simulink model "carsimplesimulink"  (R2022b)
settings: Solver=FixedStepAuto  StartTime=0.0  StopTime=inf  FixedStep=0.05  RelTol=1e-3
libraries: robotlib x7
settings Model: Creator=sprinkle  LastModifiedBy=sprinkle
settings OptimizationCC: EnhancedBackFolding=on  PassReuseOutputArgsAs=Individual arguments  ZeroExternalMemoryAtStartup=off  ZeroInternalMemoryAtStartup=off  MaxStackSize=64  OptimizeBlockOrder=speed  DifferentSizesBufferReuse=on  OptimizationCustomize=off  EfficientTunableParamExpr=on
settings DebuggingCC: ParameterTunabilityLossMsg=error
settings HardwareCC: ProdBitPerPointer=32  ProdBitPerSizeT=32  ProdBitPerPtrDiffT=32  ProdLargestAtomicFloat=None  ProdIntDivRoundTo=Undefined  ProdEndianess=Unspecified  ProdWordSize=32  ProdHWDeviceType=Generic->Unspecified (assume 32-bit Generic)
settings SFSimCC: MATLABDynamicMemAlloc=off
settings RTWCC: Description=Embedded Coder  SystemTargetFile=ert.tlc  HardwareBoard=Robot Operating System (ROS)  TLCOptions="-aInlineSetEventsForThisBaseRateFcn=TLC_FALSE -aSuppressMultiTaskScheduler=TLC_FALSE  -aRateBasedStepFcn=0"  TemplateMakefile=ert_default_tmf  Toolchain=Catkin  TargetLang=C++
settings CodeAppCC: ForceParamTrailComments=on  IgnoreCustomStorageClasses=off  OperatorAnnotations=on  SimulinkDataObjDesc=on  SFDataObjDesc=on  InsertBlockDesc=on
settings ERTTargetCC: SupportContinuousTime=on

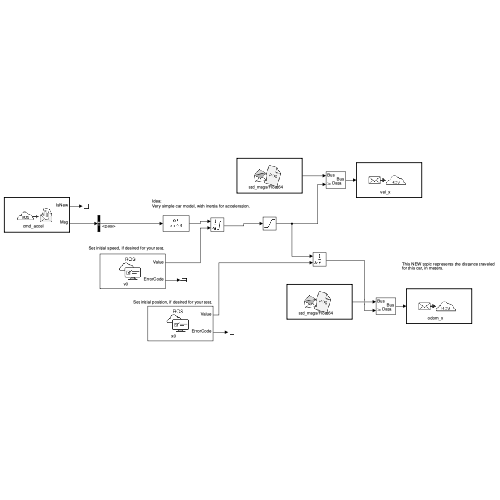
[thumbnail: Simulink's stored preview of the top-level diagram]
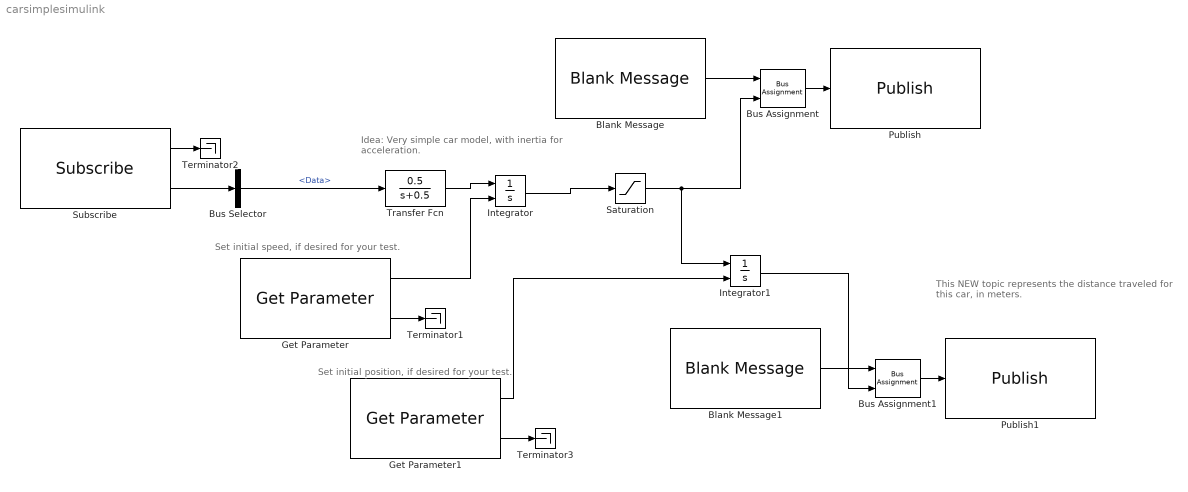
== system carsimplesimulink ==
  note: This NEW topic represents the distance traveled
      | for this car, in meters.
  note: Set initial speed, if desired for your test.
  note: Idea:
      | Very simple car model, with inertia for acceleration.
  note: Set initial position, if desired for your test.
  Blank Message : robotlib/Blank Message  messageClass=Message  entityType=std_msgs/Float64  messageType=std_msgs/Float64  SampleTime=inf  legacyBusStruct=off
      settings: LibrarySourceBlock=roslib/ROS/Blank Message
  Blank Message1 : robotlib/Blank Message  messageClass=Message  entityType=std_msgs/Float64  messageType=std_msgs/Float64  SampleTime=inf  legacyBusStruct=off
      settings: LibrarySourceBlock=roslib/ROS/Blank Message
  Bus Assignment : BusAssignment  AssignedSignals=Data
  Bus Assignment1 : BusAssignment  AssignedSignals=Data
  Bus Selector : BusSelector  OutputSignals=Data
  Get Parameter : robotlib/Get Parameter  ParameterSource=Specify your own  ParameterName=v0  ParameterType=double  ParameterMaxArrayLength=16  ParameterInitialValue=0.0  SampleTime=-1  ShowErrorCodeOutput=on  ModelName=carsimplesimulink  BlockId=ParamGet_carsimplesimulink_31
      settings: LibrarySourceBlock=roslib/ROS/Get Parameter
  Get Parameter1 : robotlib/Get Parameter  ParameterSource=Specify your own  ParameterName=x0  ParameterType=double  ParameterMaxArrayLength=16  ParameterInitialValue=0.0  SampleTime=-1  ShowErrorCodeOutput=on  ModelName=carsimplesimulink  BlockId=ParamGet_carsimplesimulink_37
      settings: LibrarySourceBlock=roslib/ROS/Get Parameter
  Integrator : Integrator  InitialConditionSource=external  LimitOutput=on  UpperSaturationLimit=40  LowerSaturationLimit=0
  Integrator1 : Integrator  InitialConditionSource=external
  Publish : robotlib/Publish  topicSource=Specify your own  topic=vel_x  messageType=std_msgs/Float64  legacyBusStruct=off  messageQueueLength=1
      settings: LibrarySourceBlock=roslib/ROS/Publish
  Publish1 : robotlib/Publish  topicSource=Specify your own  topic=odom_x  messageType=std_msgs/Float64  legacyBusStruct=off  messageQueueLength=1
      settings: LibrarySourceBlock=roslib/ROS/Publish
  Saturation : Saturate  UpperLimit=40  LowerLimit=0
  Subscribe : robotlib/Subscribe  topicSource=Specify your own  topic=cmd_accel  messageType=std_msgs/Float64  SampleTime=-1  legacyBusStruct=off  messageQueueLength=1
      settings: LibrarySourceBlock=roslib/ROS/Subscribe
  Terminator1 : Terminator
  Terminator2 : Terminator
  Terminator3 : Terminator
  Transfer Fcn : TransferFcn  Numerator=[0.5]  Denominator=[1 0.5]
  wires:
  Bus Selector/1 -> Transfer Fcn/1  "<Data>"
  Transfer Fcn/1 -> Integrator/1
  Subscribe/1 -> Terminator2/1
  Integrator/1 -> Saturation/1
  Blank Message/1 -> Bus Assignment/1
  Bus Assignment/1 -> Publish/1
  Subscribe/2 -> Bus Selector/1
  Saturation/1 -> Integrator1/1, Bus Assignment/2
  Get Parameter/1 -> Integrator/2
  Get Parameter/2 -> Terminator1/1
  Blank Message1/1 -> Bus Assignment1/1
  Bus Assignment1/1 -> Publish1/1
  Integrator1/1 -> Bus Assignment1/2
  Get Parameter1/2 -> Terminator3/1
  Get Parameter1/1 -> Integrator1/2
